simulink library "calcBankAngle_cl"  (R2020a)
settings: Solver=VariableStepAuto  StartTime=0.0  StopTime=10.0  RelTol=1e-3
libraries: VectorMagnitude_ul x3, findClosetPt_tgtPt_SlipAngle x1
settings Model: Creator=Ayaz  LastModifiedBy=Ayaz

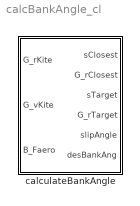
== system calcBankAngle_cl ==
  calculateBankAngle : Subsystem  mask{PW=60, PH=28, PE=30, L1=0.05, initialPathParam=0, kiteMass=0}
      mask prompts: PW "Path width [deg]"; PH "Path height [deg]"; PE "Path mean elevation [deg]"; L1 "Normalized target forward length"; initialPathParam "Initial path parameter [rad]"; kiteMass "Kite mass [kg]"
      mask TypeOptions PW: findClosetPt_tgtPt_SlipAngle/PW
      mask TypeOptions PH: findClosetPt_tgtPt_SlipAngle/PH
      mask TypeOptions PE: findClosetPt_tgtPt_SlipAngle/PE
      mask TypeOptions L1: findClosetPt_tgtPt_SlipAngle/L1

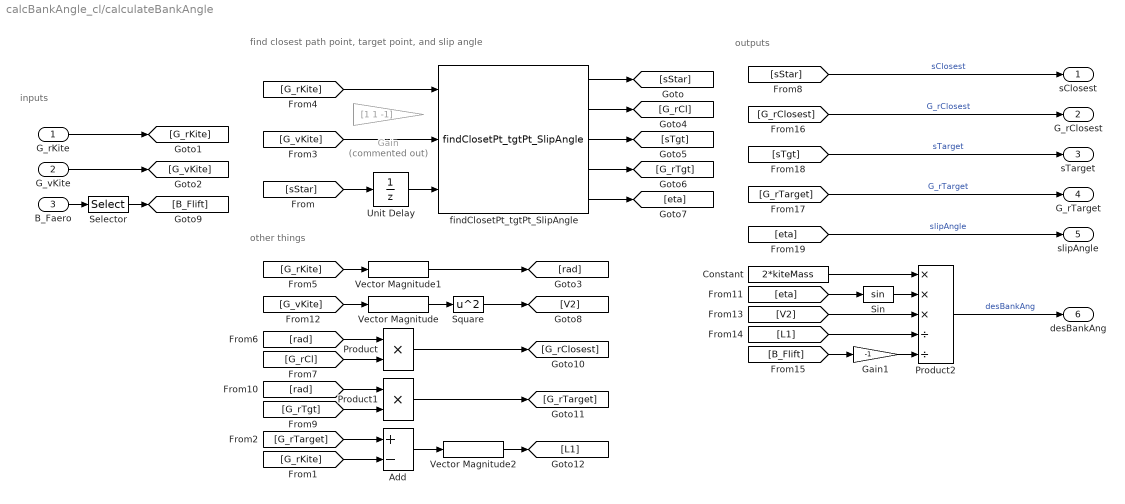
== system calcBankAngle_cl/calculateBankAngle ==
  note: find closest path point, target point, and slip angle
  note: outputs
  note: other things
  note: inputs
  G_rKite : Inport
  G_vKite : Inport  Port=2
  B_Faero : Inport  Port=3
  Add : Sum  Inputs=+-
  Constant : Constant  Value=2*kiteMass
  Gain : Gain  Commented=on  Gain=[1 1 -1]
  Gain1 : Gain  Gain=-1
  Product : Product
  Product1 : Product
  Product2 : Product  Inputs=***//
  Selector : Selector  InputPortWidth=3  IndexOptions=Index vector (dialog)  Indices=3  OutputSizes=1
  Sin : Trigonometry
  Square : Math  Operator=square  SaturateOnIntegerOverflow=on
  Unit Delay : UnitDelay  InitialCondition=initialPathParam  SampleTime=-1  HasFrameUpgradeWarning=on
  Vector Magnitude : VectorMagnitude_ul/Vector Magnitude  SystemSampleTime=-1  Latency=0  AutoFrameSizeCalculation=off
  Vector Magnitude1 : VectorMagnitude_ul/Vector Magnitude  SystemSampleTime=-1  Latency=0  AutoFrameSizeCalculation=off
  Vector Magnitude2 : VectorMagnitude_ul/Vector Magnitude  SystemSampleTime=-1  Latency=0  AutoFrameSizeCalculation=off
  findClosetPt_tgtPt_SlipAngle : findClosetPt_tgtPt_SlipAngle/findClosetPt_tgtPt_SlipAngle  PW=PW  PH=PH  PE=PE  L1=L1
  sClosest : Outport
  G_rClosest : Outport  Port=2
  sTarget : Outport  Port=3
  G_rTarget : Outport  Port=4
  slipAngle : Outport  Port=5
  desBankAng : Outport  Port=6
  wires:
  G_vKite/1 -> [G_vKite]
  G_rKite/1 -> [G_rKite]
  findClosetPt_tgtPt_SlipAngle/1 -> [sStar]
  [sStar] -> Unit Delay/1
  Unit Delay/1 -> findClosetPt_tgtPt_SlipAngle/3
  [G_vKite] -> findClosetPt_tgtPt_SlipAngle/2
  [G_rKite] -> findClosetPt_tgtPt_SlipAngle/1
  [G_rKite] -> Vector Magnitude1/1
  findClosetPt_tgtPt_SlipAngle/2 -> [G_rCl]
  [rad] -> Product/1
  [G_rCl] -> Product/2
  [sStar] -> sClosest/1  "sClosest"
  findClosetPt_tgtPt_SlipAngle/3 -> [sTgt]
  findClosetPt_tgtPt_SlipAngle/4 -> [G_rTgt]
  [G_rTgt] -> Product1/2
  [rad] -> Product1/1
  findClosetPt_tgtPt_SlipAngle/5 -> [eta]
  Vector Magnitude1/1 -> [rad]
  [eta] -> Sin/1
  [G_vKite] -> Vector Magnitude/1
  Vector Magnitude/1 -> Square/1
  Square/1 -> [V2]
  Product/1 -> [G_rClosest]
  Product1/1 -> [G_rTarget]
  [G_rKite] -> Add/2
  [G_rTarget] -> Add/1
  Add/1 -> Vector Magnitude2/1
  Vector Magnitude2/1 -> [L1]
  Sin/1 -> Product2/2
  Constant/1 -> Product2/1
  [V2] -> Product2/3
  [L1] -> Product2/4
  [B_Flift] -> Gain1/1
  [G_rClosest] -> G_rClosest/1  "G_rClosest"
  [G_rTarget] -> G_rTarget/1  "G_rTarget"
  [sTgt] -> sTarget/1  "sTarget"
  [eta] -> slipAngle/1  "slipAngle"
  Product2/1 -> desBankAng/1  "desBankAng"
  B_Faero/1 -> Selector/1
  Selector/1 -> [B_Flift]
  Gain1/1 -> Product2/5
